simulink model "new_analog_loopback_q4"  (R2015a)
settings: Solver=FixedStepDiscrete  StartTime=0.0  StopTime=inf  FixedStep=timestep  RelTol=1e-3
values from neighbouring files (symbols this model uses):
  frequency = 100    [lab1.m]
  rad = 12566    [lab1.m]    (also in old_ish.m = mean(v_radii))
libraries: slrtlib x5, xpcquanserlib x4
settings Model: SimulationMode=external  CovSFcnEnable=off  Creator=Venkatraman  LastModifiedBy=jms6
settings SolverCC: EnableConcurrentExecution=on
settings OptimizationCC: BlockReduction=off  OptimizeBlockIOStorage=off  BufferReuse=off  GlobalBufferReuse=off  ExpressionFolding=off  LocalBlockOutputs=off
settings DebuggingCC: SolverPrmCheckMsg=warning
settings HardwareCC: ProdIntDivRoundTo=Zero  ProdEndianess=LittleEndian  ProdLongLongMode=on  ProdHWDeviceType=Generic->32-bit x86 compatible  TargetLongLongMode=on  TargetIntDivRoundTo=Zero  TargetEndianess=LittleEndian  TargetHWDeviceType=MATLAB Host
settings RTWCC: SystemTargetFile=slrt.tlc  TemplateMakefile=slrt_default_tmf  Description=Simulink Real-Time  RTWVerbose=off  RTWCompilerOptimization=on
settings SimulinkRealTimeCC: GeneratePreprocessorConditionals=Disable all

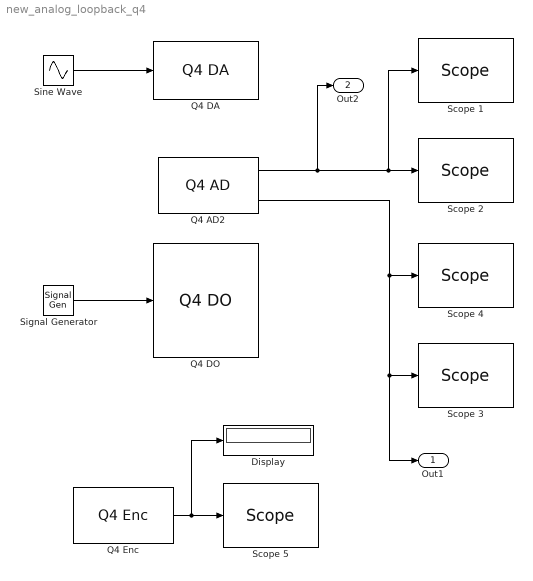
== system new_analog_loopback_q4 ==
  Display : Display
  Q4 AD2 : xpcquanserlib/A//D/Q4 AD  channel=[1 2]  sampleTime=timestep  slot=-1
  "Q4 DA " : xpcquanserlib/D//A/Q4 DA   channel=[1]  range=[-5]  simul=off  reset=[1]  initValue=[0]  sampleTime=timestep  slot=-1
  "Q4 DO " : xpcquanserlib/Digital Output/Q4 DO   channel=[2]  reset=[1]  initValue=[0]  sampleTime=timestep  slot=-1
  "Q4 Enc " : xpcquanserlib/Incremental Encoder/Q4 Enc   channel=[2]  initialCount=[0]  prescale=[1]  quadrature=[1]  mode=[0]  synchronousIndex=[0]  indexPolarity=[0]  preserveCounts=[0]  sampleTime=.001  slot=-1
  Scope 1 : slrtlib/Displays and Logging/Scope   scopeno=1  scopetype=Host  autostart=on  viewmode=Graphical redraw  formatstr='%15.6f'  grid=on  ylimits=[0,0]  nosamples=samples  noprepostsamples=0  interleave=decimation  triggermode=Software triggering  triggersignal=1  trigsignalfromport=off  triggerlevel=0.0  triggerslope=Either  triggerscope=1  triggersample=0  filename=data.dat  mode=Lazy  writesize=512  autorestart=off  dynamicfilemode=off  maxwritefilesize=512*1024^2
  Scope 2 : slrtlib/Displays and Logging/Scope   scopeno=2  scopetype=Target  autostart=on  viewmode=Graphical rolling  formatstr='%15.6f'  grid=on  ylimits=[-1,1]  nosamples=samples  noprepostsamples=0  interleave=decimation  triggermode=FreeRun  triggersignal=1  trigsignalfromport=off  triggerlevel=0.0  triggerslope=Either  triggerscope=1  triggersample=0  filename=data.dat  mode=Lazy  writesize=512  autorestart=off  dynamicfilemode=off  maxwritefilesize=512*1024^2
  Scope 3 : slrtlib/Displays and Logging/Scope   scopeno=3  scopetype=Target  autostart=on  viewmode=Graphical rolling  formatstr='%15.6f'  grid=on  ylimits=[-1,1]  nosamples=samples  noprepostsamples=0  interleave=decimation  triggermode=FreeRun  triggersignal=1  trigsignalfromport=off  triggerlevel=0.0  triggerslope=Either  triggerscope=1  triggersample=0  filename=data.dat  mode=Lazy  writesize=512  autorestart=off  dynamicfilemode=off  maxwritefilesize=512*1024^2
  Scope 4 : slrtlib/Displays and Logging/Scope   scopeno=4  scopetype=Host  autostart=on  viewmode=Graphical redraw  formatstr='%15.6f'  grid=on  ylimits=[0,0]  nosamples=samples  noprepostsamples=0  interleave=decimation  triggermode=Software triggering  triggersignal=1  trigsignalfromport=off  triggerlevel=0.0  triggerslope=Either  triggerscope=1  triggersample=0  filename=data.dat  mode=Lazy  writesize=512  autorestart=off  dynamicfilemode=off  maxwritefilesize=512*1024^2
  Scope 5 : slrtlib/Displays and Logging/Scope   scopeno=5  scopetype=Target  autostart=on  viewmode=Graphical rolling  formatstr='%15.6f'  grid=on  ylimits=[-1,1]  nosamples=samples  noprepostsamples=0  interleave=decimation  triggermode=FreeRun  triggersignal=1  trigsignalfromport=off  triggerlevel=0.0  triggerslope=Either  triggerscope=1  triggersample=0  filename=data.dat  mode=Lazy  writesize=512  autorestart=off  dynamicfilemode=off  maxwritefilesize=512*1024^2
  Signal Generator : SignalGenerator  WaveForm=square  Frequency=frequency
  Sine Wave : Sin  Frequency=rad  SampleTime=0
  Out1 : Outport
  Out2 : Outport  Port=2
  wires:
  Sine Wave/1 -> "Q4 DA "/1
  Q4 AD2/2 -> Scope 4/1, Scope 3/1, Out1/1
  Q4 AD2/1 -> Out2/1, Scope 2/1, Scope 1/1
  Signal Generator/1 -> "Q4 DO "/1
  "Q4 Enc "/1 -> Display/1, Scope 5/1
